simulink model "RC_devresi_bang_bang_kontrol"  (Simulink 10.1)
settings: Solver=FixedStepAuto  StartTime=0.0  StopTime=stopTime  FixedStep=T  RelTol=1e-3
values from neighbouring files (symbols this model uses):
  A = 10000    [init_RC_devresi_bang_bang_kontrol.m]    (also in init_araba_hiz_kontrol.m = [0 1; 0 -b/m]; init_araba_hiz_on_off_kontrol.m = [0 1; 0 -b/m]; init_araba_hiz_pid_kontrol.m = [0 1; 0 -b/m]; init_araba_pozisyon_bang_bang_kontrol.m = [0 1; 0 -b/m])
  C = 1e-4    (= 0.0001)    [init_RC_devresi.m]    (also in init_RC_devresi_bang_bang_kontrol.m; init_araba_hiz_kontrol.m = [0 1]; init_araba_hiz_on_off_kontrol.m = [0 1]; init_araba_hiz_pid_kontrol.m = [0 1])
  r = 5    [init_RC_devresi_bang_bang_kontrol.m]    (also in init_araba_hiz_kontrol.m = 90; init_araba_hiz_on_off_kontrol.m = 90; init_araba_hiz_pid_kontrol.m = 90; init_araba_pozisyon_bang_bang_kontrol.m = 1000)
  R = 1000    [init_RC_devresi.m]    (also in init_RC_devresi_bang_bang_kontrol.m)
  V0 = 0    [init_RC_devresi.m]    (also in init_RC_devresi_bang_bang_kontrol.m)
settings Model: Creator=TULPAR  LastModifiedBy=TULPAR
settings DataIOCC: SaveFormat=Dataset  SaveOutput=off  ReturnWorkspaceOutputs=on
settings OptimizationCC: LifeSpan=auto
settings DebuggingCC: UnderspecifiedInitializationDetection=Simplified  MergeDetectMultiDrivingBlocksExec=error  SFUnexpectedBacktrackingDiag=error  SFNoUnconditionalDefaultTransitionDiag=error  SFExecutionAtInitializationDiag=warning  ArithmeticOperatorsInVariantConditions=error
settings HardwareCC: ProdBitPerPointer=64  ProdBitPerSizeT=64  ProdBitPerPtrDiffT=64  ProdLargestAtomicFloat=Float  ProdIntDivRoundTo=Zero  ProdEndianess=LittleEndian  ProdWordSize=64  ProdHWDeviceType=Intel->x86-64 (Windows64)
settings ModelReferenceCC: PropagateSignalLabelsOutOfModel=on
settings SFSimCC: SimUseLocalCustomCode=on  CustomCodeUndefinedFunction=FilterOut
settings RTWCC: RTWUseLocalCustomCode=on
settings CodeAppCC: StateflowObjectComments=off
settings GRTTargetCC: TargetLangStandard=C99 (ISO)  CombineOutputUpdateFcns=on  GRTInterface=off
settings ConfigComp: CovMetricSettings=dwe  CovHtmlReporting=off  CovSaveCumulativeToWorkspaceVar=off  CovSaveSingleToWorkspaceVar=off  CovExternalEMLEnable=on

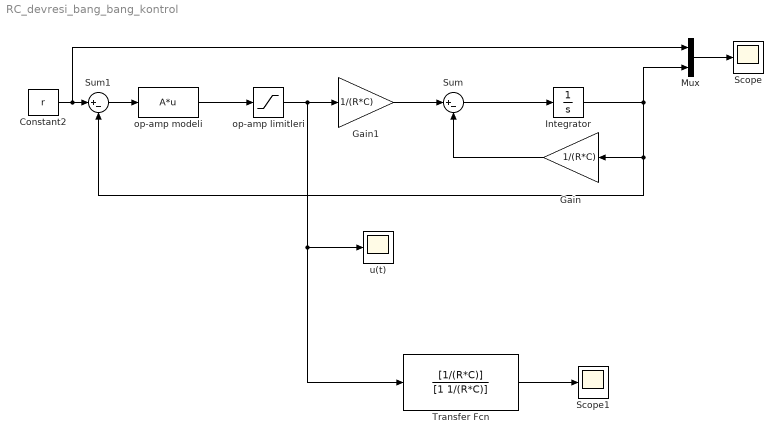
== system RC_devresi_bang_bang_kontrol ==
  Constant2 : Constant  Value=r
  Gain : Gain  Gain=1/(R*C)
  Gain1 : Gain  Gain=1/(R*C)
  Integrator : Integrator  InitialCondition=V0
  Mux : Mux  Inputs=2
  Scope : Scope
  Scope1 : Scope
  Sum : Sum  Inputs=|+-
  Sum1 : Sum  Inputs=|+-
  Transfer Fcn : TransferFcn  Numerator=[1/(R*C)]  Denominator=[1 1/(R*C)]
  op-amp limitleri : Saturate  UpperLimit=12  LowerLimit=-12
  op-amp modeli : Fcn  Expr=A*u
  u(t) : Scope
  wires:
  Gain1/1 -> Sum/1
  Integrator/1 -> Gain/1, Sum1/2, Mux/2
  Gain/1 -> Sum/2
  Sum/1 -> Integrator/1
  op-amp limitleri/1 -> u(t)/1, Transfer Fcn/1, Gain1/1
  Transfer Fcn/1 -> Scope1/1
  op-amp modeli/1 -> op-amp limitleri/1
  Mux/1 -> Scope/1
  Sum1/1 -> op-amp modeli/1
  Constant2/1 -> Mux/1, Sum1/1
